simulink model "EDoS_model"  (R2020b)
settings: Solver=VariableStepAuto  StartTime=0.0  StopTime=200000  RelTol=1e-3
values from neighbouring files (symbols this model uses):
  attackRate = 0    [init_model.m]
  initialLoopWaitTime = 1000    [init_model.m]    (also in plot_results.m = 50)
  lowerUtilThreshold = 50    [init_model.m]    (also in plot_results.m)
  maxCores = 35    [init_model.m]    (also in plot_results.m)
  routineRate = 4    [init_model.m]    (also in plot_results.m)
  scalingLoopDelay = 500    [init_model.m]    (also in plot_results.m = 5)
  scalingStep = 2    [init_model.m]    (also in plot_results.m)
  upperUtilThreshold = 80    [init_model.m]    (also in plot_results.m)
undefined symbols (not defined in the file or in its folder): m, n
libraries: simulink x2
(part 3 of 3)

== system EDoS_model/Multiprocessor_scalable_system/Balancer ==
  blocked : Inport
  fillOf : Inport  Port=2
  MATLAB Function1 : MATLAB Function  TreatAsAtomicUnit=on
  Message Send : Send  OutputPortMessageModes=m
  SelectedPort : Outport
  wires:
  MATLAB Function1/1(selectedPort) -> Message Send/1
  blocked/1 -> MATLAB Function1/1(blocked)
  Message Send/1 -> SelectedPort/1
  fillOf/1 -> MATLAB Function1/2(fillOf)

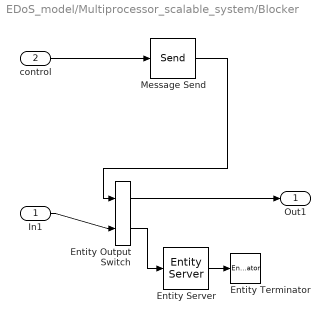
== system EDoS_model/Multiprocessor_scalable_system/Blocker ==
  In1 : Inport
  control : Inport  Port=2
  Entity Output Switch : EntityOutputSwitch  InputPortMessageModes=m,m  OutputPortMessageModes=m,m  SwitchingCriterion=From control port  SwitchAttributeName=Attribute1  InitialPortSelection=2
      settings: InputPortMap=u0,u1
  Entity Server : EntityServer  InputPortMessageModes=m  OutputPortMessageModes=m  Capacity=1  ServiceTimeValue=inf
  Entity Terminator : EntityTerminator  InputPortMessageModes=m
  Message Send : Send  OutputPortMessageModes=m
  Out1 : Outport
  wires:
  In1/1 -> Entity Output Switch/2
  Entity Output Switch/1 -> Out1/1
  Entity Output Switch/2 -> Entity Server/1
  Entity Server/1 -> Entity Terminator/1
  Message Send/1 -> Entity Output Switch/1
  control/1 -> Message Send/1

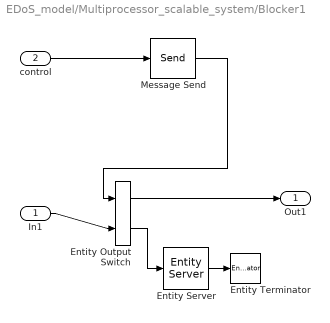
== system EDoS_model/Multiprocessor_scalable_system/Blocker1 ==
  In1 : Inport
  control : Inport  Port=2
  Entity Output Switch : EntityOutputSwitch  InputPortMessageModes=m,m  OutputPortMessageModes=m,m  SwitchingCriterion=From control port  SwitchAttributeName=Attribute1  InitialPortSelection=2
      settings: InputPortMap=u0,u1
  Entity Server : EntityServer  InputPortMessageModes=m  OutputPortMessageModes=m  Capacity=1  ServiceTimeValue=inf
  Entity Terminator : EntityTerminator  InputPortMessageModes=m
  Message Send : Send  OutputPortMessageModes=m
  Out1 : Outport
  wires:
  In1/1 -> Entity Output Switch/2
  Entity Output Switch/1 -> Out1/1
  Entity Output Switch/2 -> Entity Server/1
  Entity Server/1 -> Entity Terminator/1
  Message Send/1 -> Entity Output Switch/1
  control/1 -> Message Send/1

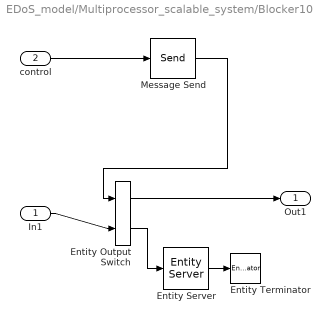
== system EDoS_model/Multiprocessor_scalable_system/Blocker10 ==
  In1 : Inport
  control : Inport  Port=2
  Entity Output Switch : EntityOutputSwitch  InputPortMessageModes=m,m  OutputPortMessageModes=m,m  SwitchingCriterion=From control port  SwitchAttributeName=Attribute1  InitialPortSelection=2
      settings: InputPortMap=u0,u1
  Entity Server : EntityServer  InputPortMessageModes=m  OutputPortMessageModes=m  Capacity=1  ServiceTimeValue=inf
  Entity Terminator : EntityTerminator  InputPortMessageModes=m
  Message Send : Send  OutputPortMessageModes=m
  Out1 : Outport
  wires:
  In1/1 -> Entity Output Switch/2
  Entity Output Switch/1 -> Out1/1
  Entity Output Switch/2 -> Entity Server/1
  Entity Server/1 -> Entity Terminator/1
  Message Send/1 -> Entity Output Switch/1
  control/1 -> Message Send/1

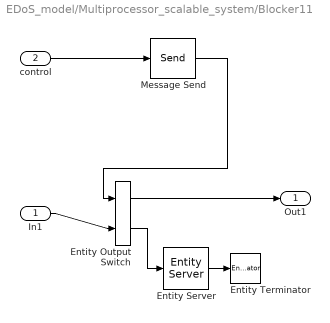
== system EDoS_model/Multiprocessor_scalable_system/Blocker11 ==
  In1 : Inport
  control : Inport  Port=2
  Entity Output Switch : EntityOutputSwitch  InputPortMessageModes=m,m  OutputPortMessageModes=m,m  SwitchingCriterion=From control port  SwitchAttributeName=Attribute1  InitialPortSelection=2
      settings: InputPortMap=u0,u1
  Entity Server : EntityServer  InputPortMessageModes=m  OutputPortMessageModes=m  Capacity=1  ServiceTimeValue=inf
  Entity Terminator : EntityTerminator  InputPortMessageModes=m
  Message Send : Send  OutputPortMessageModes=m
  Out1 : Outport
  wires:
  In1/1 -> Entity Output Switch/2
  Entity Output Switch/1 -> Out1/1
  Entity Output Switch/2 -> Entity Server/1
  Entity Server/1 -> Entity Terminator/1
  Message Send/1 -> Entity Output Switch/1
  control/1 -> Message Send/1

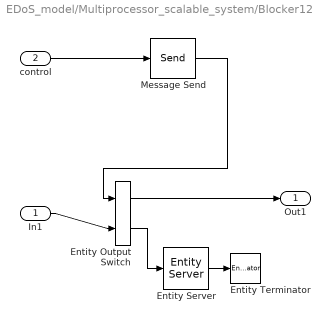
== system EDoS_model/Multiprocessor_scalable_system/Blocker12 ==
  In1 : Inport
  control : Inport  Port=2
  Entity Output Switch : EntityOutputSwitch  InputPortMessageModes=m,m  OutputPortMessageModes=m,m  SwitchingCriterion=From control port  SwitchAttributeName=Attribute1  InitialPortSelection=2
      settings: InputPortMap=u0,u1
  Entity Server : EntityServer  InputPortMessageModes=m  OutputPortMessageModes=m  Capacity=1  ServiceTimeValue=inf
  Entity Terminator : EntityTerminator  InputPortMessageModes=m
  Message Send : Send  OutputPortMessageModes=m
  Out1 : Outport
  wires:
  In1/1 -> Entity Output Switch/2
  Entity Output Switch/1 -> Out1/1
  Entity Output Switch/2 -> Entity Server/1
  Entity Server/1 -> Entity Terminator/1
  Message Send/1 -> Entity Output Switch/1
  control/1 -> Message Send/1

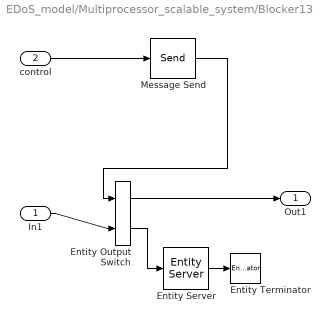
== system EDoS_model/Multiprocessor_scalable_system/Blocker13 ==
  In1 : Inport
  control : Inport  Port=2
  Entity Output Switch : EntityOutputSwitch  InputPortMessageModes=m,m  OutputPortMessageModes=m,m  SwitchingCriterion=From control port  SwitchAttributeName=Attribute1  InitialPortSelection=2
      settings: InputPortMap=u0,u1
  Entity Server : EntityServer  InputPortMessageModes=m  OutputPortMessageModes=m  Capacity=1  ServiceTimeValue=inf
  Entity Terminator : EntityTerminator  InputPortMessageModes=m
  Message Send : Send  OutputPortMessageModes=m
  Out1 : Outport
  wires:
  In1/1 -> Entity Output Switch/2
  Entity Output Switch/1 -> Out1/1
  Entity Output Switch/2 -> Entity Server/1
  Entity Server/1 -> Entity Terminator/1
  Message Send/1 -> Entity Output Switch/1
  control/1 -> Message Send/1

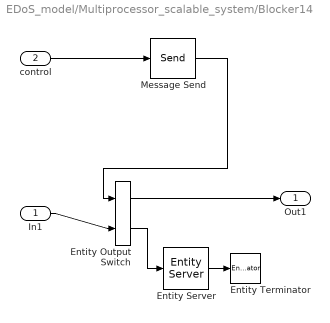
== system EDoS_model/Multiprocessor_scalable_system/Blocker14 ==
  In1 : Inport
  control : Inport  Port=2
  Entity Output Switch : EntityOutputSwitch  InputPortMessageModes=m,m  OutputPortMessageModes=m,m  SwitchingCriterion=From control port  SwitchAttributeName=Attribute1  InitialPortSelection=2
      settings: InputPortMap=u0,u1
  Entity Server : EntityServer  InputPortMessageModes=m  OutputPortMessageModes=m  Capacity=1  ServiceTimeValue=inf
  Entity Terminator : EntityTerminator  InputPortMessageModes=m
  Message Send : Send  OutputPortMessageModes=m
  Out1 : Outport
  wires:
  In1/1 -> Entity Output Switch/2
  Entity Output Switch/1 -> Out1/1
  Entity Output Switch/2 -> Entity Server/1
  Entity Server/1 -> Entity Terminator/1
  Message Send/1 -> Entity Output Switch/1
  control/1 -> Message Send/1

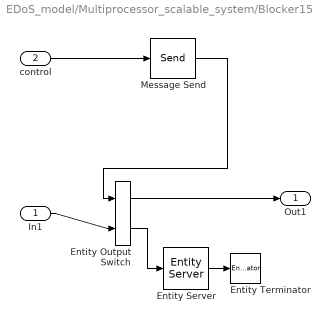
== system EDoS_model/Multiprocessor_scalable_system/Blocker15 ==
  In1 : Inport
  control : Inport  Port=2
  Entity Output Switch : EntityOutputSwitch  InputPortMessageModes=m,m  OutputPortMessageModes=m,m  SwitchingCriterion=From control port  SwitchAttributeName=Attribute1  InitialPortSelection=2
      settings: InputPortMap=u0,u1
  Entity Server : EntityServer  InputPortMessageModes=m  OutputPortMessageModes=m  Capacity=1  ServiceTimeValue=inf
  Entity Terminator : EntityTerminator  InputPortMessageModes=m
  Message Send : Send  OutputPortMessageModes=m
  Out1 : Outport
  wires:
  In1/1 -> Entity Output Switch/2
  Entity Output Switch/1 -> Out1/1
  Entity Output Switch/2 -> Entity Server/1
  Entity Server/1 -> Entity Terminator/1
  Message Send/1 -> Entity Output Switch/1
  control/1 -> Message Send/1

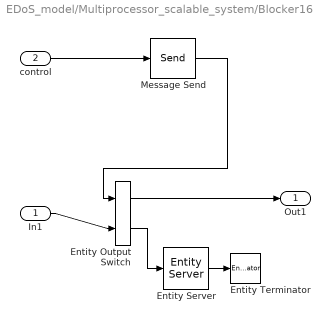
== system EDoS_model/Multiprocessor_scalable_system/Blocker16 ==
  In1 : Inport
  control : Inport  Port=2
  Entity Output Switch : EntityOutputSwitch  InputPortMessageModes=m,m  OutputPortMessageModes=m,m  SwitchingCriterion=From control port  SwitchAttributeName=Attribute1  InitialPortSelection=2
      settings: InputPortMap=u0,u1
  Entity Server : EntityServer  InputPortMessageModes=m  OutputPortMessageModes=m  Capacity=1  ServiceTimeValue=inf
  Entity Terminator : EntityTerminator  InputPortMessageModes=m
  Message Send : Send  OutputPortMessageModes=m
  Out1 : Outport
  wires:
  In1/1 -> Entity Output Switch/2
  Entity Output Switch/1 -> Out1/1
  Entity Output Switch/2 -> Entity Server/1
  Entity Server/1 -> Entity Terminator/1
  Message Send/1 -> Entity Output Switch/1
  control/1 -> Message Send/1

== system EDoS_model/Multiprocessor_scalable_system/Blocker17 ==
  In1 : Inport
  control : Inport  Port=2
  Entity Output Switch : EntityOutputSwitch  InputPortMessageModes=m,m  OutputPortMessageModes=m,m  SwitchingCriterion=From control port  SwitchAttributeName=Attribute1  InitialPortSelection=2
      settings: InputPortMap=u0,u1
  Entity Server : EntityServer  InputPortMessageModes=m  OutputPortMessageModes=m  Capacity=1  ServiceTimeValue=inf
  Entity Terminator : EntityTerminator  InputPortMessageModes=m
  Message Send : Send  OutputPortMessageModes=m
  Out1 : Outport
  wires:
  In1/1 -> Entity Output Switch/2
  Entity Output Switch/1 -> Out1/1
  Entity Output Switch/2 -> Entity Server/1
  Entity Server/1 -> Entity Terminator/1
  Message Send/1 -> Entity Output Switch/1
  control/1 -> Message Send/1

== system EDoS_model/Multiprocessor_scalable_system/Blocker18 ==
  In1 : Inport
  control : Inport  Port=2
  Entity Output Switch : EntityOutputSwitch  InputPortMessageModes=m,m  OutputPortMessageModes=m,m  SwitchingCriterion=From control port  SwitchAttributeName=Attribute1  InitialPortSelection=2
      settings: InputPortMap=u0,u1
  Entity Server : EntityServer  InputPortMessageModes=m  OutputPortMessageModes=m  Capacity=1  ServiceTimeValue=inf
  Entity Terminator : EntityTerminator  InputPortMessageModes=m
  Message Send : Send  OutputPortMessageModes=m
  Out1 : Outport
  wires:
  In1/1 -> Entity Output Switch/2
  Entity Output Switch/1 -> Out1/1
  Entity Output Switch/2 -> Entity Server/1
  Entity Server/1 -> Entity Terminator/1
  Message Send/1 -> Entity Output Switch/1
  control/1 -> Message Send/1

== system EDoS_model/Multiprocessor_scalable_system/Blocker19 ==
  In1 : Inport
  control : Inport  Port=2
  Entity Output Switch : EntityOutputSwitch  InputPortMessageModes=m,m  OutputPortMessageModes=m,m  SwitchingCriterion=From control port  SwitchAttributeName=Attribute1  InitialPortSelection=2
      settings: InputPortMap=u0,u1
  Entity Server : EntityServer  InputPortMessageModes=m  OutputPortMessageModes=m  Capacity=1  ServiceTimeValue=inf
  Entity Terminator : EntityTerminator  InputPortMessageModes=m
  Message Send : Send  OutputPortMessageModes=m
  Out1 : Outport
  wires:
  In1/1 -> Entity Output Switch/2
  Entity Output Switch/1 -> Out1/1
  Entity Output Switch/2 -> Entity Server/1
  Entity Server/1 -> Entity Terminator/1
  Message Send/1 -> Entity Output Switch/1
  control/1 -> Message Send/1

== system EDoS_model/Multiprocessor_scalable_system/Blocker2 ==
  In1 : Inport
  control : Inport  Port=2
  Entity Output Switch : EntityOutputSwitch  InputPortMessageModes=m,m  OutputPortMessageModes=m,m  SwitchingCriterion=From control port  SwitchAttributeName=Attribute1  InitialPortSelection=2
      settings: InputPortMap=u0,u1
  Entity Server : EntityServer  InputPortMessageModes=m  OutputPortMessageModes=m  Capacity=1  ServiceTimeValue=inf
  Entity Terminator : EntityTerminator  InputPortMessageModes=m
  Message Send : Send  OutputPortMessageModes=m
  Out1 : Outport
  wires:
  In1/1 -> Entity Output Switch/2
  Entity Output Switch/1 -> Out1/1
  Entity Output Switch/2 -> Entity Server/1
  Entity Server/1 -> Entity Terminator/1
  Message Send/1 -> Entity Output Switch/1
  control/1 -> Message Send/1

== system EDoS_model/Multiprocessor_scalable_system/Blocker20 ==
  In1 : Inport
  control : Inport  Port=2
  Entity Output Switch : EntityOutputSwitch  InputPortMessageModes=m,m  OutputPortMessageModes=m,m  SwitchingCriterion=From control port  SwitchAttributeName=Attribute1  InitialPortSelection=2
      settings: InputPortMap=u0,u1
  Entity Server : EntityServer  InputPortMessageModes=m  OutputPortMessageModes=m  Capacity=1  ServiceTimeValue=inf
  Entity Terminator : EntityTerminator  InputPortMessageModes=m
  Message Send : Send  OutputPortMessageModes=m
  Out1 : Outport
  wires:
  In1/1 -> Entity Output Switch/2
  Entity Output Switch/1 -> Out1/1
  Entity Output Switch/2 -> Entity Server/1
  Entity Server/1 -> Entity Terminator/1
  Message Send/1 -> Entity Output Switch/1
  control/1 -> Message Send/1

== system EDoS_model/Multiprocessor_scalable_system/Blocker21 ==
  In1 : Inport
  control : Inport  Port=2
  Entity Output Switch : EntityOutputSwitch  InputPortMessageModes=m,m  OutputPortMessageModes=m,m  SwitchingCriterion=From control port  SwitchAttributeName=Attribute1  InitialPortSelection=2
      settings: InputPortMap=u0,u1
  Entity Server : EntityServer  InputPortMessageModes=m  OutputPortMessageModes=m  Capacity=1  ServiceTimeValue=inf
  Entity Terminator : EntityTerminator  InputPortMessageModes=m
  Message Send : Send  OutputPortMessageModes=m
  Out1 : Outport
  wires:
  In1/1 -> Entity Output Switch/2
  Entity Output Switch/1 -> Out1/1
  Entity Output Switch/2 -> Entity Server/1
  Entity Server/1 -> Entity Terminator/1
  Message Send/1 -> Entity Output Switch/1
  control/1 -> Message Send/1

== system EDoS_model/Multiprocessor_scalable_system/Blocker22 ==
  In1 : Inport
  control : Inport  Port=2
  Entity Output Switch : EntityOutputSwitch  InputPortMessageModes=m,m  OutputPortMessageModes=m,m  SwitchingCriterion=From control port  SwitchAttributeName=Attribute1  InitialPortSelection=2
      settings: InputPortMap=u0,u1
  Entity Server : EntityServer  InputPortMessageModes=m  OutputPortMessageModes=m  Capacity=1  ServiceTimeValue=inf
  Entity Terminator : EntityTerminator  InputPortMessageModes=m
  Message Send : Send  OutputPortMessageModes=m
  Out1 : Outport
  wires:
  In1/1 -> Entity Output Switch/2
  Entity Output Switch/1 -> Out1/1
  Entity Output Switch/2 -> Entity Server/1
  Entity Server/1 -> Entity Terminator/1
  Message Send/1 -> Entity Output Switch/1
  control/1 -> Message Send/1

== system EDoS_model/Multiprocessor_scalable_system/Blocker23 ==
  In1 : Inport
  control : Inport  Port=2
  Entity Output Switch : EntityOutputSwitch  InputPortMessageModes=m,m  OutputPortMessageModes=m,m  SwitchingCriterion=From control port  SwitchAttributeName=Attribute1  InitialPortSelection=2
      settings: InputPortMap=u0,u1
  Entity Server : EntityServer  InputPortMessageModes=m  OutputPortMessageModes=m  Capacity=1  ServiceTimeValue=inf
  Entity Terminator : EntityTerminator  InputPortMessageModes=m
  Message Send : Send  OutputPortMessageModes=m
  Out1 : Outport
  wires:
  In1/1 -> Entity Output Switch/2
  Entity Output Switch/1 -> Out1/1
  Entity Output Switch/2 -> Entity Server/1
  Entity Server/1 -> Entity Terminator/1
  Message Send/1 -> Entity Output Switch/1
  control/1 -> Message Send/1

== system EDoS_model/Multiprocessor_scalable_system/Blocker24 ==
  In1 : Inport
  control : Inport  Port=2
  Entity Output Switch : EntityOutputSwitch  InputPortMessageModes=m,m  OutputPortMessageModes=m,m  SwitchingCriterion=From control port  SwitchAttributeName=Attribute1  InitialPortSelection=2
      settings: InputPortMap=u0,u1
  Entity Server : EntityServer  InputPortMessageModes=m  OutputPortMessageModes=m  Capacity=1  ServiceTimeValue=inf
  Entity Terminator : EntityTerminator  InputPortMessageModes=m
  Message Send : Send  OutputPortMessageModes=m
  Out1 : Outport
  wires:
  In1/1 -> Entity Output Switch/2
  Entity Output Switch/1 -> Out1/1
  Entity Output Switch/2 -> Entity Server/1
  Entity Server/1 -> Entity Terminator/1
  Message Send/1 -> Entity Output Switch/1
  control/1 -> Message Send/1

== system EDoS_model/Multiprocessor_scalable_system/Blocker25 ==
  In1 : Inport
  control : Inport  Port=2
  Entity Output Switch : EntityOutputSwitch  InputPortMessageModes=m,m  OutputPortMessageModes=m,m  SwitchingCriterion=From control port  SwitchAttributeName=Attribute1  InitialPortSelection=2
      settings: InputPortMap=u0,u1
  Entity Server : EntityServer  InputPortMessageModes=m  OutputPortMessageModes=m  Capacity=1  ServiceTimeValue=inf
  Entity Terminator : EntityTerminator  InputPortMessageModes=m
  Message Send : Send  OutputPortMessageModes=m
  Out1 : Outport
  wires:
  In1/1 -> Entity Output Switch/2
  Entity Output Switch/1 -> Out1/1
  Entity Output Switch/2 -> Entity Server/1
  Entity Server/1 -> Entity Terminator/1
  Message Send/1 -> Entity Output Switch/1
  control/1 -> Message Send/1

== system EDoS_model/Multiprocessor_scalable_system/Blocker26 ==
  In1 : Inport
  control : Inport  Port=2
  Entity Output Switch : EntityOutputSwitch  InputPortMessageModes=m,m  OutputPortMessageModes=m,m  SwitchingCriterion=From control port  SwitchAttributeName=Attribute1  InitialPortSelection=2
      settings: InputPortMap=u0,u1
  Entity Server : EntityServer  InputPortMessageModes=m  OutputPortMessageModes=m  Capacity=1  ServiceTimeValue=inf
  Entity Terminator : EntityTerminator  InputPortMessageModes=m
  Message Send : Send  OutputPortMessageModes=m
  Out1 : Outport
  wires:
  In1/1 -> Entity Output Switch/2
  Entity Output Switch/1 -> Out1/1
  Entity Output Switch/2 -> Entity Server/1
  Entity Server/1 -> Entity Terminator/1
  Message Send/1 -> Entity Output Switch/1
  control/1 -> Message Send/1

== system EDoS_model/Multiprocessor_scalable_system/Blocker27 ==
  In1 : Inport
  control : Inport  Port=2
  Entity Output Switch : EntityOutputSwitch  InputPortMessageModes=m,m  OutputPortMessageModes=m,m  SwitchingCriterion=From control port  SwitchAttributeName=Attribute1  InitialPortSelection=2
      settings: InputPortMap=u0,u1
  Entity Server : EntityServer  InputPortMessageModes=m  OutputPortMessageModes=m  Capacity=1  ServiceTimeValue=inf
  Entity Terminator : EntityTerminator  InputPortMessageModes=m
  Message Send : Send  OutputPortMessageModes=m
  Out1 : Outport
  wires:
  In1/1 -> Entity Output Switch/2
  Entity Output Switch/1 -> Out1/1
  Entity Output Switch/2 -> Entity Server/1
  Entity Server/1 -> Entity Terminator/1
  Message Send/1 -> Entity Output Switch/1
  control/1 -> Message Send/1

== system EDoS_model/Multiprocessor_scalable_system/Blocker28 ==
  In1 : Inport
  control : Inport  Port=2
  Entity Output Switch : EntityOutputSwitch  InputPortMessageModes=m,m  OutputPortMessageModes=m,m  SwitchingCriterion=From control port  SwitchAttributeName=Attribute1  InitialPortSelection=2
      settings: InputPortMap=u0,u1
  Entity Server : EntityServer  InputPortMessageModes=m  OutputPortMessageModes=m  Capacity=1  ServiceTimeValue=inf
  Entity Terminator : EntityTerminator  InputPortMessageModes=m
  Message Send : Send  OutputPortMessageModes=m
  Out1 : Outport
  wires:
  In1/1 -> Entity Output Switch/2
  Entity Output Switch/1 -> Out1/1
  Entity Output Switch/2 -> Entity Server/1
  Entity Server/1 -> Entity Terminator/1
  Message Send/1 -> Entity Output Switch/1
  control/1 -> Message Send/1

== system EDoS_model/Multiprocessor_scalable_system/Blocker29 ==
  In1 : Inport
  control : Inport  Port=2
  Entity Output Switch : EntityOutputSwitch  InputPortMessageModes=m,m  OutputPortMessageModes=m,m  SwitchingCriterion=From control port  SwitchAttributeName=Attribute1  InitialPortSelection=2
      settings: InputPortMap=u0,u1
  Entity Server : EntityServer  InputPortMessageModes=m  OutputPortMessageModes=m  Capacity=1  ServiceTimeValue=inf
  Entity Terminator : EntityTerminator  InputPortMessageModes=m
  Message Send : Send  OutputPortMessageModes=m
  Out1 : Outport
  wires:
  In1/1 -> Entity Output Switch/2
  Entity Output Switch/1 -> Out1/1
  Entity Output Switch/2 -> Entity Server/1
  Entity Server/1 -> Entity Terminator/1
  Message Send/1 -> Entity Output Switch/1
  control/1 -> Message Send/1

== system EDoS_model/Multiprocessor_scalable_system/Blocker3 ==
  In1 : Inport
  control : Inport  Port=2
  Entity Output Switch : EntityOutputSwitch  InputPortMessageModes=m,m  OutputPortMessageModes=m,m  SwitchingCriterion=From control port  SwitchAttributeName=Attribute1  InitialPortSelection=2
      settings: InputPortMap=u0,u1
  Entity Server : EntityServer  InputPortMessageModes=m  OutputPortMessageModes=m  Capacity=1  ServiceTimeValue=inf
  Entity Terminator : EntityTerminator  InputPortMessageModes=m
  Message Send : Send  OutputPortMessageModes=m
  Out1 : Outport
  wires:
  In1/1 -> Entity Output Switch/2
  Entity Output Switch/1 -> Out1/1
  Entity Output Switch/2 -> Entity Server/1
  Entity Server/1 -> Entity Terminator/1
  Message Send/1 -> Entity Output Switch/1
  control/1 -> Message Send/1

== system EDoS_model/Multiprocessor_scalable_system/Blocker30 ==
  In1 : Inport
  control : Inport  Port=2
  Entity Output Switch : EntityOutputSwitch  InputPortMessageModes=m,m  OutputPortMessageModes=m,m  SwitchingCriterion=From control port  SwitchAttributeName=Attribute1  InitialPortSelection=2
      settings: InputPortMap=u0,u1
  Entity Server : EntityServer  InputPortMessageModes=m  OutputPortMessageModes=m  Capacity=1  ServiceTimeValue=inf
  Entity Terminator : EntityTerminator  InputPortMessageModes=m
  Message Send : Send  OutputPortMessageModes=m
  Out1 : Outport
  wires:
  In1/1 -> Entity Output Switch/2
  Entity Output Switch/1 -> Out1/1
  Entity Output Switch/2 -> Entity Server/1
  Entity Server/1 -> Entity Terminator/1
  Message Send/1 -> Entity Output Switch/1
  control/1 -> Message Send/1

== system EDoS_model/Multiprocessor_scalable_system/Blocker31 ==
  In1 : Inport
  control : Inport  Port=2
  Entity Output Switch : EntityOutputSwitch  InputPortMessageModes=m,m  OutputPortMessageModes=m,m  SwitchingCriterion=From control port  SwitchAttributeName=Attribute1  InitialPortSelection=2
      settings: InputPortMap=u0,u1
  Entity Server : EntityServer  InputPortMessageModes=m  OutputPortMessageModes=m  Capacity=1  ServiceTimeValue=inf
  Entity Terminator : EntityTerminator  InputPortMessageModes=m
  Message Send : Send  OutputPortMessageModes=m
  Out1 : Outport
  wires:
  In1/1 -> Entity Output Switch/2
  Entity Output Switch/1 -> Out1/1
  Entity Output Switch/2 -> Entity Server/1
  Entity Server/1 -> Entity Terminator/1
  Message Send/1 -> Entity Output Switch/1
  control/1 -> Message Send/1

== system EDoS_model/Multiprocessor_scalable_system/Blocker32 ==
  In1 : Inport
  control : Inport  Port=2
  Entity Output Switch : EntityOutputSwitch  InputPortMessageModes=m,m  OutputPortMessageModes=m,m  SwitchingCriterion=From control port  SwitchAttributeName=Attribute1  InitialPortSelection=2
      settings: InputPortMap=u0,u1
  Entity Server : EntityServer  InputPortMessageModes=m  OutputPortMessageModes=m  Capacity=1  ServiceTimeValue=inf
  Entity Terminator : EntityTerminator  InputPortMessageModes=m
  Message Send : Send  OutputPortMessageModes=m
  Out1 : Outport
  wires:
  In1/1 -> Entity Output Switch/2
  Entity Output Switch/1 -> Out1/1
  Entity Output Switch/2 -> Entity Server/1
  Entity Server/1 -> Entity Terminator/1
  Message Send/1 -> Entity Output Switch/1
  control/1 -> Message Send/1

== system EDoS_model/Multiprocessor_scalable_system/Blocker33 ==
  In1 : Inport
  control : Inport  Port=2
  Entity Output Switch : EntityOutputSwitch  InputPortMessageModes=m,m  OutputPortMessageModes=m,m  SwitchingCriterion=From control port  SwitchAttributeName=Attribute1  InitialPortSelection=2
      settings: InputPortMap=u0,u1
  Entity Server : EntityServer  InputPortMessageModes=m  OutputPortMessageModes=m  Capacity=1  ServiceTimeValue=inf
  Entity Terminator : EntityTerminator  InputPortMessageModes=m
  Message Send : Send  OutputPortMessageModes=m
  Out1 : Outport
  wires:
  In1/1 -> Entity Output Switch/2
  Entity Output Switch/1 -> Out1/1
  Entity Output Switch/2 -> Entity Server/1
  Entity Server/1 -> Entity Terminator/1
  Message Send/1 -> Entity Output Switch/1
  control/1 -> Message Send/1

== system EDoS_model/Multiprocessor_scalable_system/Blocker34 ==
  In1 : Inport
  control : Inport  Port=2
  Entity Output Switch : EntityOutputSwitch  InputPortMessageModes=m,m  OutputPortMessageModes=m,m  SwitchingCriterion=From control port  SwitchAttributeName=Attribute1  InitialPortSelection=2
      settings: InputPortMap=u0,u1
  Entity Server : EntityServer  InputPortMessageModes=m  OutputPortMessageModes=m  Capacity=1  ServiceTimeValue=inf
  Entity Terminator : EntityTerminator  InputPortMessageModes=m
  Message Send : Send  OutputPortMessageModes=m
  Out1 : Outport
  wires:
  In1/1 -> Entity Output Switch/2
  Entity Output Switch/1 -> Out1/1
  Entity Output Switch/2 -> Entity Server/1
  Entity Server/1 -> Entity Terminator/1
  Message Send/1 -> Entity Output Switch/1
  control/1 -> Message Send/1

== system EDoS_model/Multiprocessor_scalable_system/Blocker4 ==
  In1 : Inport
  control : Inport  Port=2
  Entity Output Switch : EntityOutputSwitch  InputPortMessageModes=m,m  OutputPortMessageModes=m,m  SwitchingCriterion=From control port  SwitchAttributeName=Attribute1  InitialPortSelection=2
      settings: InputPortMap=u0,u1
  Entity Server : EntityServer  InputPortMessageModes=m  OutputPortMessageModes=m  Capacity=1  ServiceTimeValue=inf
  Entity Terminator : EntityTerminator  InputPortMessageModes=m
  Message Send : Send  OutputPortMessageModes=m
  Out1 : Outport
  wires:
  In1/1 -> Entity Output Switch/2
  Entity Output Switch/1 -> Out1/1
  Entity Output Switch/2 -> Entity Server/1
  Entity Server/1 -> Entity Terminator/1
  Message Send/1 -> Entity Output Switch/1
  control/1 -> Message Send/1

== system EDoS_model/Multiprocessor_scalable_system/Blocker5 ==
  In1 : Inport
  control : Inport  Port=2
  Entity Output Switch : EntityOutputSwitch  InputPortMessageModes=m,m  OutputPortMessageModes=m,m  SwitchingCriterion=From control port  SwitchAttributeName=Attribute1  InitialPortSelection=2
      settings: InputPortMap=u0,u1
  Entity Server : EntityServer  InputPortMessageModes=m  OutputPortMessageModes=m  Capacity=1  ServiceTimeValue=inf
  Entity Terminator : EntityTerminator  InputPortMessageModes=m
  Message Send : Send  OutputPortMessageModes=m
  Out1 : Outport
  wires:
  In1/1 -> Entity Output Switch/2
  Entity Output Switch/1 -> Out1/1
  Entity Output Switch/2 -> Entity Server/1
  Entity Server/1 -> Entity Terminator/1
  Message Send/1 -> Entity Output Switch/1
  control/1 -> Message Send/1

== system EDoS_model/Multiprocessor_scalable_system/Blocker6 ==
  In1 : Inport
  control : Inport  Port=2
  Entity Output Switch : EntityOutputSwitch  InputPortMessageModes=m,m  OutputPortMessageModes=m,m  SwitchingCriterion=From control port  SwitchAttributeName=Attribute1  InitialPortSelection=2
      settings: InputPortMap=u0,u1
  Entity Server : EntityServer  InputPortMessageModes=m  OutputPortMessageModes=m  Capacity=1  ServiceTimeValue=inf
  Entity Terminator : EntityTerminator  InputPortMessageModes=m
  Message Send : Send  OutputPortMessageModes=m
  Out1 : Outport
  wires:
  In1/1 -> Entity Output Switch/2
  Entity Output Switch/1 -> Out1/1
  Entity Output Switch/2 -> Entity Server/1
  Entity Server/1 -> Entity Terminator/1
  Message Send/1 -> Entity Output Switch/1
  control/1 -> Message Send/1

== system EDoS_model/Multiprocessor_scalable_system/Blocker7 ==
  In1 : Inport
  control : Inport  Port=2
  Entity Output Switch : EntityOutputSwitch  InputPortMessageModes=m,m  OutputPortMessageModes=m,m  SwitchingCriterion=From control port  SwitchAttributeName=Attribute1  InitialPortSelection=2
      settings: InputPortMap=u0,u1
  Entity Server : EntityServer  InputPortMessageModes=m  OutputPortMessageModes=m  Capacity=1  ServiceTimeValue=inf
  Entity Terminator : EntityTerminator  InputPortMessageModes=m
  Message Send : Send  OutputPortMessageModes=m
  Out1 : Outport
  wires:
  In1/1 -> Entity Output Switch/2
  Entity Output Switch/1 -> Out1/1
  Entity Output Switch/2 -> Entity Server/1
  Entity Server/1 -> Entity Terminator/1
  Message Send/1 -> Entity Output Switch/1
  control/1 -> Message Send/1

== system EDoS_model/Multiprocessor_scalable_system/Blocker8 ==
  In1 : Inport
  control : Inport  Port=2
  Entity Output Switch : EntityOutputSwitch  InputPortMessageModes=m,m  OutputPortMessageModes=m,m  SwitchingCriterion=From control port  SwitchAttributeName=Attribute1  InitialPortSelection=2
      settings: InputPortMap=u0,u1
  Entity Server : EntityServer  InputPortMessageModes=m  OutputPortMessageModes=m  Capacity=1  ServiceTimeValue=inf
  Entity Terminator : EntityTerminator  InputPortMessageModes=m
  Message Send : Send  OutputPortMessageModes=m
  Out1 : Outport
  wires:
  In1/1 -> Entity Output Switch/2
  Entity Output Switch/1 -> Out1/1
  Entity Output Switch/2 -> Entity Server/1
  Entity Server/1 -> Entity Terminator/1
  Message Send/1 -> Entity Output Switch/1
  control/1 -> Message Send/1

== system EDoS_model/Multiprocessor_scalable_system/Blocker9 ==
  In1 : Inport
  control : Inport  Port=2
  Entity Output Switch : EntityOutputSwitch  InputPortMessageModes=m,m  OutputPortMessageModes=m,m  SwitchingCriterion=From control port  SwitchAttributeName=Attribute1  InitialPortSelection=2
      settings: InputPortMap=u0,u1
  Entity Server : EntityServer  InputPortMessageModes=m  OutputPortMessageModes=m  Capacity=1  ServiceTimeValue=inf
  Entity Terminator : EntityTerminator  InputPortMessageModes=m
  Message Send : Send  OutputPortMessageModes=m
  Out1 : Outport
  wires:
  In1/1 -> Entity Output Switch/2
  Entity Output Switch/1 -> Out1/1
  Entity Output Switch/2 -> Entity Server/1
  Entity Server/1 -> Entity Terminator/1
  Message Send/1 -> Entity Output Switch/1
  control/1 -> Message Send/1

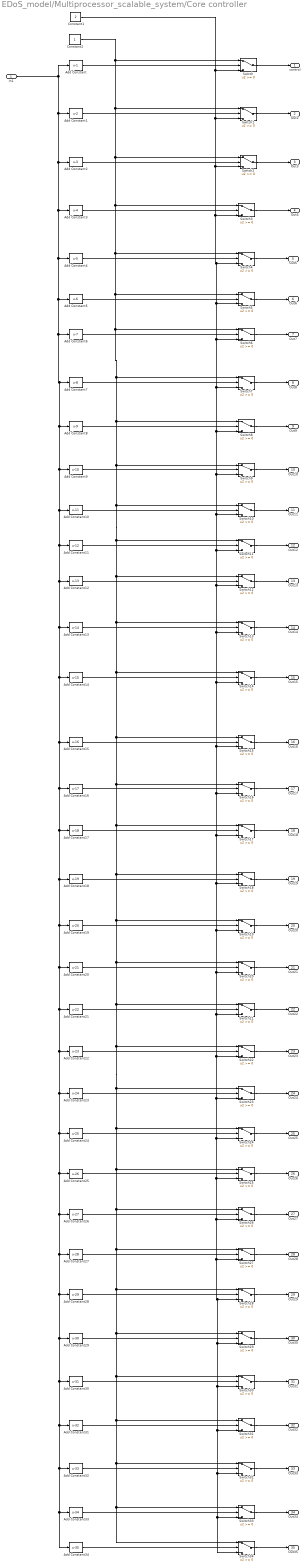
== system EDoS_model/Multiprocessor_scalable_system/Core controller ==
  In1 : Inport
  Add Constant : Bias  Bias=-1
  Add Constant1 : Bias  Bias=-2
  Add Constant10 : Bias  Bias=-11
  Add Constant11 : Bias  Bias=-12
  Add Constant12 : Bias  Bias=-13
  Add Constant13 : Bias  Bias=-14
  Add Constant14 : Bias  Bias=-15
  Add Constant15 : Bias  Bias=-16
  Add Constant16 : Bias  Bias=-17
  Add Constant17 : Bias  Bias=-18
  Add Constant18 : Bias  Bias=-19
  Add Constant19 : Bias  Bias=-20
  Add Constant2 : Bias  Bias=-3
  Add Constant20 : Bias  Bias=-21
  Add Constant21 : Bias  Bias=-22
  Add Constant22 : Bias  Bias=-23
  Add Constant23 : Bias  Bias=-24
  Add Constant24 : Bias  Bias=-25
  Add Constant25 : Bias  Bias=-26
  Add Constant26 : Bias  Bias=-27
  Add Constant27 : Bias  Bias=-28
  Add Constant28 : Bias  Bias=-29
  Add Constant29 : Bias  Bias=-30
  Add Constant3 : Bias  Bias=-4
  Add Constant30 : Bias  Bias=-31
  Add Constant31 : Bias  Bias=-32
  Add Constant32 : Bias  Bias=-33
  Add Constant33 : Bias  Bias=-34
  Add Constant34 : Bias  Bias=-35
  Add Constant4 : Bias  Bias=-5
  Add Constant5 : Bias  Bias=-6
  Add Constant6 : Bias  Bias=-7
  Add Constant7 : Bias  Bias=-8
  Add Constant8 : Bias  Bias=-9
  Add Constant9 : Bias  Bias=-10
  Constant1 : Constant  Value=2
  Constant2 : Constant
  Switch{,1..34} (35 alike) : Switch
  control : Outport
  Out2 : Outport  Port=2
  Out3 : Outport  Port=3
  Out4 : Outport  Port=4
  Out5 : Outport  Port=5
  Out6 : Outport  Port=6
  Out7 : Outport  Port=7
  Out8 : Outport  Port=8
  Out9 : Outport  Port=9
  Out10 : Outport  Port=10
  Out11 : Outport  Port=11
  Out12 : Outport  Port=12
  Out13 : Outport  Port=13
  Out14 : Outport  Port=14
  Out15 : Outport  Port=15
  Out16 : Outport  Port=16
  Out17 : Outport  Port=17
  Out18 : Outport  Port=18
  Out19 : Outport  Port=19
  Out20 : Outport  Port=20
  Out21 : Outport  Port=21
  Out22 : Outport  Port=22
  Out23 : Outport  Port=23
  Out24 : Outport  Port=24
  Out25 : Outport  Port=25
  Out26 : Outport  Port=26
  Out27 : Outport  Port=27
  Out28 : Outport  Port=28
  Out29 : Outport  Port=29
  Out30 : Outport  Port=30
  Out31 : Outport  Port=31
  Out32 : Outport  Port=32
  Out33 : Outport  Port=33
  Out34 : Outport  Port=34
  Out35 : Outport  Port=35
  wires:
  Switch/1 -> control/1
  Switch1/1 -> Out2/1
  Switch2/1 -> Out3/1
  Switch3/1 -> Out4/1
  Switch4/1 -> Out5/1
  Add Constant/1 -> Switch/2
  Add Constant1/1 -> Switch1/2
  Add Constant2/1 -> Switch2/2
  Add Constant3/1 -> Switch3/2
  Add Constant4/1 -> Switch4/2
  Add Constant5/1 -> Switch5/2
  Add Constant6/1 -> Switch6/2
  Switch5/1 -> Out6/1
  Switch6/1 -> Out7/1
  Add Constant7/1 -> Switch7/2
  Switch7/1 -> Out8/1
  Switch8/1 -> Out9/1
  Add Constant8/1 -> Switch8/2
  Add Constant9/1 -> Switch9/2
  Add Constant10/1 -> Switch10/2
  Switch9/1 -> Out10/1
  Switch10/1 -> Out11/1
  Add Constant11/1 -> Switch11/2
  Switch11/1 -> Out12/1
  Add Constant12/1 -> Switch12/2
  Switch12/1 -> Out13/1
  Add Constant13/1 -> Switch13/2
  Switch13/1 -> Out14/1
  Add Constant14/1 -> Switch14/2
  Add Constant15/1 -> Switch15/2
  Switch15/1 -> Out16/1
  Switch14/1 -> Out15/1
  Add Constant16/1 -> Switch16/2
  Switch16/1 -> Out17/1
  Add Constant17/1 -> Switch17/2
  Switch17/1 -> Out18/1
  Add Constant18/1 -> Switch18/2
  Switch18/1 -> Out19/1
  Add Constant19/1 -> Switch19/2
  Switch19/1 -> Out20/1
  Add Constant20/1 -> Switch20/2
  Switch20/1 -> Out21/1
  Add Constant21/1 -> Switch21/2
  Switch21/1 -> Out22/1
  Add Constant22/1 -> Switch22/2
  Switch22/1 -> Out23/1
  Add Constant23/1 -> Switch23/2
  Switch23/1 -> Out24/1
  Add Constant24/1 -> Switch24/2
  Switch24/1 -> Out25/1
  Add Constant25/1 -> Switch25/2
  Switch25/1 -> Out26/1
  Add Constant26/1 -> Switch26/2
  Switch26/1 -> Out27/1
  Add Constant27/1 -> Switch27/2
  Switch27/1 -> Out28/1
  Add Constant28/1 -> Switch28/2
  Switch28/1 -> Out29/1
  Add Constant29/1 -> Switch29/2
  Switch29/1 -> Out30/1
  Add Constant30/1 -> Switch30/2
  Switch30/1 -> Out31/1
  Add Constant31/1 -> Switch31/2
  Switch31/1 -> Out32/1
  Add Constant32/1 -> Switch32/2
  Switch32/1 -> Out33/1
  Add Constant33/1 -> Switch33/2
  Switch33/1 -> Out34/1
  Switch34/1 -> Out35/1
  Add Constant34/1 -> Switch34/2
  Constant1/1 -> Switch18/3, Switch34/3, Switch33/3, Switch32/3, Switch31/3, Switch30/3, Switch29/3, Switch28/3, Switch27/3, Switch26/3, Switch25/3, Switch24/3, Switch23/3, Switch22/3, Switch21/3, Switch20/3, Switch19/3, Switch17/3, Switch16/3, Switch15/3, Switch14/3, Switch13/3, Switch12/3, Switch11/3, Switch10/3, Switch9/3, Switch8/3, Switch7/3, Switch6/3, Switch5/3, Switch4/3, Switch3/3, Switch2/3, Switch1/3, Switch/3
  In1/1 -> Add Constant6/1, Add Constant34/1, Add Constant33/1, Add Constant32/1, Add Constant31/1, Add Constant30/1, Add Constant29/1, Add Constant28/1, Add Constant27/1, Add Constant26/1, Add Constant25/1, Add Constant24/1, Add Constant23/1, Add Constant22/1, Add Constant21/1, Add Constant20/1, Add Constant19/1, Add Constant18/1, Add Constant17/1, Add Constant16/1, Add Constant15/1, Add Constant14/1, Add Constant13/1, Add Constant12/1, Add Constant11/1, Add Constant10/1, Add Constant9/1, Add Constant8/1, Add Constant7/1, Add Constant5/1, Add Constant4/1, Add Constant3/1, Add Constant2/1, Add Constant1/1, Add Constant/1
  Constant2/1 -> Switch/1, Switch1/1, Switch2/1, Switch3/1, Switch4/1, Switch5/1, Switch6/1, Switch7/1, Switch8/1, Switch9/1, Switch10/1, Switch11/1, Switch12/1, Switch13/1, Switch14/1, Switch15/1, Switch16/1, Switch17/1, Switch18/1, Switch19/1, Switch20/1, Switch21/1, Switch22/1, Switch23/1, Switch24/1, Switch25/1, Switch26/1, Switch27/1, Switch28/1, Switch29/1, Switch30/1, Switch31/1, Switch32/1, Switch34/1, Switch33/1

== matlab function EDoS_model/randPoissionTrafic ==
  data: dt output; attackRate input; routineRate input
function dt = randPoissionTrafic(attackRate, routineRate)

    lambda = 10;
    c = 0.767 - 3.36/lambda;
    beta = pi/sqrt(3.0*lambda);
    alpha = beta*lambda;
    k = log(c) - lambda - log(beta);

    while true
        u = rand(1);
	    x = (alpha - log((1.0 - u)/u))/beta;
	    n = floor(x + 0.5);
	    if (n < 0)
		    continue;
        end    
	    v = rand(1);
	    y = alpha - beta*x;
	    lhs = y + log(v/(1.0 + exp(y))^2);
	    rhs = k + n*log(lambda) - log(factorial(n));
	    if (lhs <= rhs)
		    break;
        end    
    end  
    dt = n /(routineRate + attackRate);

== matlab function EDoS_model/Multiprocessor_scalable_system/MATLAB Function ==
  data: upperThresh input; lowerThresh input; maxCores input; scalingStep input; coresNow input; util input
function fcn(upperThresh, lowerThresh, maxCores, scalingStep, coresNow, util)
      
  eml.extrinsic('num2str');
  coder.extrinsic('set_param');
  if util > 0
    utilPerCore = util / coresNow;
    if(utilPerCore > upperThresh && coresNow < maxCores)
        coresNew = round(coresNow + scalingStep);
        if (coresNew > maxCores)
           coresNew = maxCores; 
        end    
        p = num2str(coresNew);
        set_param('EDoS_model/Multiprocessor_scalable_system/Gain1', 'Gain', p); 
    end    

    if(utilPerCore < lowerThresh && coresNow > 1)
        coresNew = round(coresNow - scalingStep);
        if (coresNew < 1)
           coresNew = 1; 
        end 
        p = num2str(coresNew);
        set_param('EDoS_model/Multiprocessor_scalable_system/Gain1', 'Gain', p); 
    end   
  end

== matlab function EDoS_model/Multiprocessor_scalable_system/Balancer/MATLAB Function1 ==
  data: blocked input; fillOf input; selectedPort output
function selectedPort = balancerFunc(blocked, fillOf)
    

    unblocked = -1 * (blocked - 3) - 1;
    unblockedId = find(unblocked);
    fillOfUnblocked = fillOf(unblockedId);
    
    minPorts = find(fillOfUnblocked == min(fillOfUnblocked));
    
    n = length(minPorts) - 1;
    
    selectedPort = minPorts(round(n * rand(1) + 1));
